simulink model "SCARA"  (R2015a)
settings: Solver=ode1  StartTime=0.0  StopTime=Inf  FixedStep=0.001  RelTol=1e-3
PostLoadFcn:
  | , if any(exist('dsrtsu_mdlpostloadfcn', 'file') == [2, 3, 6]), try dsrtsu_mdlpostloadfcn('Execute', bdroot); catch fprintf('Error in PostLoadFcn (dsrtsu_mdlpostloadfcn) for model "%s":\n %s\n', bdroot, lasterr); end, end,
libraries: rtilib1104 x9
settings Model: DSRTSU_INTERNAL_RTI_VER=460  DSRTSU_INTERNAL_RTI_TYPE=rti1104  DSRTSU_INTERNAL_RTIFPGA=50  CovHtmlReporting=off  Creator=k21s1315a  LastModifiedBy=k21s1315a
settings OptimizationCC: BlockReduction=off  OptimizeBlockIOStorage=off  BufferReuse=off  GlobalBufferReuse=off  ExpressionFolding=off  LocalBlockOutputs=off
settings HardwareCC: ProdIntDivRoundTo=Zero  ProdEndianess=BigEndian  ProdHWDeviceType=Generic->Custom  TargetIntDivRoundTo=Zero  TargetEndianess=BigEndian  TargetHWDeviceType=Generic->Custom
settings RTWCC: SystemTargetFile=rti1104.tlc  MakeCommand=make_rti  TemplateMakefile=rti1104.tmf  Description=dSPACE DS1104 Hardware Platform
settings STFCustomTargetCC: GenerateSampleERTMain=off  ParMdlRefBuildCompliant=on  GeneratePreprocessorConditionals=Disable all  ERTCustomFileBanners=off  SupportNonInlinedSFcns=on  SupportVariableSizeSignals=off  MATLABClassNameForMDSCustomization=Simulink.SoftwareTarget.GRTCustomization  GRTInterface=on  SystemTargetFile=rti1104.tlc
settings GRTTargetCC: CompOptLevelCompliant=off  ConcurrentExecutionCompliant=off  CombineOutputUpdateFcns=off  MatFileLogging=off  CPPClassGenCompliant=off  GRTInterface=on  ExtModeMexFile=noextcomm

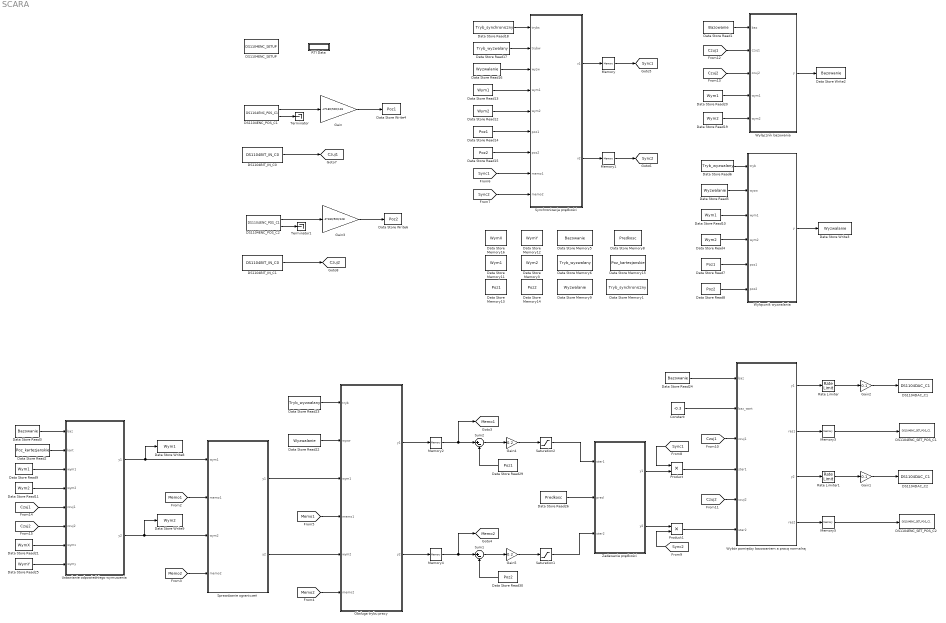
== system SCARA ==
  Constant : Constant  Value=-0.3
  DS1104BIT_IN_C0 : rtilib1104/DS1104 MASTER PPC/DS1104BIT_IN_C0  ChannelNo=0  Reserved1=[]  Reserved2=[]  Reserved3=[]  Reserved4=[]  DialogFcn=gui1104bit_in  UnitName={'DS1104BIT_IN_C'}  UnitValues={ 0 }  DSProperties=struct('RTI',struct('Version',uint32(1),'BlockType',struct('isSLSource',uint8(1),'isSLSink',uint8(0),'isHWSource',uint8(1),'isHWSink',uint8(0),'isSetup',uint8(0),'isInline',uint8(1),'isNonInline',uint8(0),'isInterrupt',uint8(0),'isChannelwise',uint8(1)),'IOBoardType','DS1104MASTER','UnitType','BIT','Identifier','BITINCH','DialogType','ML','BlockSet','NONE','SlaveProcessor','NONE'))
  DS1104BIT_IN_C1 : rtilib1104/DS1104 MASTER PPC/DS1104BIT_IN_C0  ChannelNo=1  Reserved1=[]  Reserved2=[]  Reserved3=[]  Reserved4=[]  DialogFcn=gui1104bit_in  UnitName={'DS1104BIT_IN_C'}  UnitValues={1}  DSProperties=struct('RTI',struct('Version',uint32(1),'BlockType',struct('isSLSource',uint8(1),'isSLSink',uint8(0),'isHWSource',uint8(1),'isHWSink',uint8(0),'isSetup',uint8(0),'isInline',uint8(1),'isNonInline',uint8(0),'isInterrupt',uint8(0),'isChannelwise',uint8(1)),'IOBoardType','DS1104MASTER','UnitType','BIT','Identifier','BITINCH','DialogType','ML','BlockSet','NONE','SlaveProcessor','NONE'))
  DS1104DAC_C1 : rtilib1104/DS1104 MASTER PPC/DS1104DAC_C1  ChannelNo=1  InitValue=0  TermMode=0  TermValue=0  Reserved1=[]  Reserved2=[]  Reserved3=[]  Reserved4=[]  DialogFcn=gui1104dac  UnitName={ 'DS1104DAC_C'}  UnitValues={ 1 }  DSProperties=struct('RTI',struct('Version',uint32(1),'BlockType',struct('isSLSource',uint8(0),'isSLSink',uint8(1),'isHWSource',uint8(0),'isHWSink',uint8(1),'isSetup',uint8(0),'isInline',uint8(1),'isNonInline',uint8(0),'isInterrupt',uint8(0),'isChannelwise',uint8(1)),'IOBoardType','DS1104MASTER','UnitType','DAC','Identifier','DAC','DialogType','ML','BlockSet','NONE','SlaveProcessor','NONE'))
  DS1104DAC_C2 : rtilib1104/DS1104 MASTER PPC/DS1104DAC_C1  ChannelNo=2  InitValue=0  TermMode=0  TermValue=0  Reserved1=[]  Reserved2=[]  Reserved3=[]  Reserved4=[]  DialogFcn=gui1104dac  UnitName={ 'DS1104DAC_C'}  UnitValues={2}  DSProperties=struct('RTI',struct('Version',uint32(1),'BlockType',struct('isSLSource',uint8(0),'isSLSink',uint8(1),'isHWSource',uint8(0),'isHWSink',uint8(1),'isSetup',uint8(0),'isInline',uint8(1),'isNonInline',uint8(0),'isInterrupt',uint8(0),'isChannelwise',uint8(1)),'IOBoardType','DS1104MASTER','UnitType','DAC','Identifier','DAC','DialogType','ML','BlockSet','NONE','SlaveProcessor','NONE'))
  DS1104ENC_POS_C1 : rtilib1104/DS1104 MASTER PPC/DS1104ENC_POS_C1  ChannelNo=1  PosValue=0  Reserved1=[]  Reserved2=[]  Reserved3=[]  Reserved4=[]  DialogFcn=gui1104enc_pos  UnitName={'DS1104ENC_POS_C'}  UnitValues={ 1 }  DSProperties=struct('RTI',struct('Version',uint32(1),'BlockType',struct('isSLSource',uint8(1),'isSLSink',uint8(0),'isHWSource',uint8(1),'isHWSink',uint8(0),'isSetup',uint8(0),'isInline',uint8(1),'isNonInline',uint8(0),'isInterrupt',uint8(0),'isChannelwise',uint8(1)),'IOBoardType','DS1104MASTER','UnitType','ENC','Identifier','ENCPOSCH','DialogType','ML','BlockSet','NONE','SlaveProcessor','NONE'))
  DS1104ENC_POS_C2 : rtilib1104/DS1104 MASTER PPC/DS1104ENC_POS_C1  ChannelNo=2  PosValue=0  Reserved1=[]  Reserved2=[]  Reserved3=[]  Reserved4=[]  DialogFcn=gui1104enc_pos  UnitName={'DS1104ENC_POS_C'}  UnitValues={2}  DSProperties=struct('RTI',struct('Version',uint32(1),'BlockType',struct('isSLSource',uint8(1),'isSLSink',uint8(0),'isHWSource',uint8(1),'isHWSink',uint8(0),'isSetup',uint8(0),'isInline',uint8(1),'isNonInline',uint8(0),'isInterrupt',uint8(0),'isChannelwise',uint8(1)),'IOBoardType','DS1104MASTER','UnitType','ENC','Identifier','ENCPOSCH','DialogType','ML','BlockSet','NONE','SlaveProcessor','NONE'))
  DS1104ENC_SETUP : rtilib1104/DS1104 MASTER PPC/DS1104ENC_SETUP  Reserved1=[]  Reserved2=[]  Reserved3=[]  Reserved4=[]  DialogFcn=gui1104enc_setup  UnitName={'DS1104ENC_SETUP'}  UnitValues={ [] }  DSProperties=struct('RTI',struct('Version',uint32(1),'BlockType',struct('isSLSource',uint8(0),'isSLSink',uint8(0),'isHWSource',uint8(0),'isHWSink',uint8(0),'isSetup',uint8(0),'isInline',uint8(1),'isNonInline',uint8(0),'isInterrupt',uint8(0),'isChannelwise',uint8(0)),'IOBoardType','DS1104MASTER','UnitType','ENC','Identifier','ENCSETUP','DialogType','ML','BlockSet','NONE','SlaveProcessor','NONE'))
      settings: SignalType=[0 0]
  DS1104ENC_SET_POS_C1 : rtilib1104/DS1104 MASTER PPC/DS1104ENC_SET_POS_C1  ChannelNo=1  PosValue=0  Reserved1=[]  Reserved2=[]  Reserved3=[]  Reserved4=[]  DialogFcn=gui1104enc_set_pos  UnitName={'DS1104ENC_SET_POS_C'}  UnitValues={ 1 }  DSProperties=struct('RTI',struct('Version',uint32(1),'BlockType',struct('isSLSource',uint8(0),'isSLSink',uint8(1),'isHWSource',uint8(0),'isHWSink',uint8(1),'isSetup',uint8(0),'isInline',uint8(1),'isNonInline',uint8(0),'isInterrupt',uint8(0),'isChannelwise',uint8(1)),'IOBoardType','DS1104MASTER','UnitType','ENC','Identifier','ENCRESET','DialogType','ML','BlockSet','NONE','SlaveProcessor','NONE'))
  DS1104ENC_SET_POS_C2 : rtilib1104/DS1104 MASTER PPC/DS1104ENC_SET_POS_C1  ChannelNo=2  PosValue=0  Reserved1=[]  Reserved2=[]  Reserved3=[]  Reserved4=[]  DialogFcn=gui1104enc_set_pos  UnitName={'DS1104ENC_SET_POS_C'}  UnitValues={2}  DSProperties=struct('RTI',struct('Version',uint32(1),'BlockType',struct('isSLSource',uint8(0),'isSLSink',uint8(1),'isHWSource',uint8(0),'isHWSink',uint8(1),'isSetup',uint8(0),'isInline',uint8(1),'isNonInline',uint8(0),'isInterrupt',uint8(0),'isChannelwise',uint8(1)),'IOBoardType','DS1104MASTER','UnitType','ENC','Identifier','ENCRESET','DialogType','ML','BlockSet','NONE','SlaveProcessor','NONE'))
  Data Store Memory1 : DataStoreMemory  DataStoreName=Tryb_synchroniczny  ReadBeforeWriteMsg=warning  WriteAfterWriteMsg=warning  WriteAfterReadMsg=warning
  Data Store Memory11 : DataStoreMemory  DataStoreName=Wym1  ReadBeforeWriteMsg=warning  WriteAfterWriteMsg=warning  WriteAfterReadMsg=warning
  Data Store Memory12 : DataStoreMemory  DataStoreName=WymY  ReadBeforeWriteMsg=warning  WriteAfterWriteMsg=warning  WriteAfterReadMsg=warning
  Data Store Memory13 : DataStoreMemory  DataStoreName=Poz1  ReadBeforeWriteMsg=warning  WriteAfterWriteMsg=warning  WriteAfterReadMsg=warning
  Data Store Memory14 : DataStoreMemory  DataStoreName=Poz2  ReadBeforeWriteMsg=warning  WriteAfterWriteMsg=warning  WriteAfterReadMsg=warning
  Data Store Memory15 : DataStoreMemory  DataStoreName=Poz_kartezjanskie  ReadBeforeWriteMsg=warning  WriteAfterWriteMsg=warning  WriteAfterReadMsg=warning
  Data Store Memory16 : DataStoreMemory  DataStoreName=WymX  ReadBeforeWriteMsg=warning  WriteAfterWriteMsg=warning  WriteAfterReadMsg=warning
  Data Store Memory3 : DataStoreMemory  DataStoreName=Wym2  ReadBeforeWriteMsg=warning  WriteAfterWriteMsg=warning  WriteAfterReadMsg=warning
  Data Store Memory5 : DataStoreMemory  DataStoreName=Bazowanie  ReadBeforeWriteMsg=warning  WriteAfterWriteMsg=warning  WriteAfterReadMsg=warning
  Data Store Memory6 : DataStoreMemory  DataStoreName=Tryb_wyzwalany  ReadBeforeWriteMsg=warning  WriteAfterWriteMsg=warning  WriteAfterReadMsg=warning
  Data Store Memory8 : DataStoreMemory  DataStoreName=Predkosc  ReadBeforeWriteMsg=warning  WriteAfterWriteMsg=warning  WriteAfterReadMsg=warning
  Data Store Memory9 : DataStoreMemory  DataStoreName=Wyzwalanie  ReadBeforeWriteMsg=warning  WriteAfterWriteMsg=warning  WriteAfterReadMsg=warning
  Data Store Read1 : DataStoreRead  DataStoreName=Bazowanie
  Data Store Read{9..10,13,20} (4 alike) : DataStoreRead  DataStoreName=Wym1
  Data Store Read{4,11..12,19} (4 alike) : DataStoreRead  DataStoreName=Wym2
  Data Store Read14 : DataStoreRead  DataStoreName=Poz1
  Data Store Read15 : DataStoreRead  DataStoreName=Poz2
  Data Store Read16 : DataStoreRead  DataStoreName=Wyzwalanie
  Data Store Read17 : DataStoreRead  DataStoreName=Tryb_wyzwalany
  Data Store Read18 : DataStoreRead  DataStoreName=Tryb_synchroniczny
  Data Store Read2 : DataStoreRead  DataStoreName=Poz_kartezjanskie
  Data Store Read21 : DataStoreRead  DataStoreName=WymX
  Data Store Read22 : DataStoreRead  DataStoreName=Wyzwalanie
  Data Store Read23 : DataStoreRead  DataStoreName=Tryb_wyzwalany
  Data Store Read24 : DataStoreRead  DataStoreName=Bazowanie
  Data Store Read25 : DataStoreRead  DataStoreName=WymY
  Data Store Read26 : DataStoreRead  DataStoreName=Predkosc
  Data Store Read29 : DataStoreRead  DataStoreName=Poz1
  Data Store Read3 : DataStoreRead  DataStoreName=Bazowanie
  Data Store Read30 : DataStoreRead  DataStoreName=Poz2
  Data Store Read5 : DataStoreRead  DataStoreName=Wyzwalanie
  Data Store Read6 : DataStoreRead  DataStoreName=Tryb_wyzwalany
  Data Store Read7 : DataStoreRead  DataStoreName=Poz1
  Data Store Read8 : DataStoreRead  DataStoreName=Poz2
  Data Store Write2 : DataStoreWrite  DataStoreName=Bazowanie
  Data Store Write3 : DataStoreWrite  DataStoreName=Wyzwalanie
  Data Store Write4 : DataStoreWrite  DataStoreName=Poz1
  Data Store Write6 : DataStoreWrite  DataStoreName=Poz2
  Data Store Write8 : DataStoreWrite  DataStoreName=Wym1
  Data Store Write9 : DataStoreWrite  DataStoreName=Wym2
  Gain : Gain  Gain=-2*180/500/128
  Gain1 : Gain  Gain=0.1
  Gain2 : Gain  Gain=0.1
  Gain3 : Gain  Gain=-2*180/500/128
  Gain4 : Gain  Gain=0.2
  Gain5 : Gain  Gain=0.2
  Memory{,1,3,5} (4 alike) : Memory  X0=1
  Memory2 : Memory
  Memory4 : Memory
  Obsługa trybu pracy : MATLAB Function  TreatAsAtomicUnit=on
  Product : Product
  Product1 : Product
  RTI Data : Subsystem  Tag=struct('RTIDataServer',struct('RTIDataServerVs','2','RTIModelDescription','struct(''main'',''Scara_model'',''sub'','''',''isMp'',0)'))  LoadFcn="if exist('rtidc'), try,  rtidc('DataHostBlockClbLoad', gcbh); catch, disp(['Warning: ''LoadFcn'' for RTI Data block failed: ' lasterr]); end, end,"  mask(RTI_DATA_HOST){}
      mask help:
      | RTI Data Block.
      | This block is used by RTI to store internal model-dependent data.
      | Please keep this block on the root level of the model. Deleting this block will result in data loss.
      |
      | NEVER DELETE OR COPY THIS BLOCK!
      settings: CopyFcn="if exist('rtidc'), try,  rtidc('DataHostBlockClbCopy', gcbh); catch, disp(['Warning: ''CopyFcn'' for RTI Data block failed: ' lasterr]); end, end,"  DeleteFcn="if exist('rtidc'), try,  rtidc('DataHostBlockClbDelete', gcbh); catch, disp(['Warning: ''DeleteFcn'' for RTI Data block failed: ' lasterr]); end, end,"  ModelCloseFcn="if exist('rtidc'), try,  rtidc('DataHostBlockClbModelClose', gcbh); catch, disp(['Warning: ''ModelCloseFcn'' for RTI Data block failed: ' lasterr]); end, end,"  PreSaveFcn="if exist('rtidc'), try,  rtidc('DataHostBlockClbPreSave', gcbh); catch, disp(['Warning: ''PreSaveFcn'' for RTI Data block failed: ' lasterr]); end, end,"  PostSaveFcn="if exist('rtidc'), try,  rtidc('DataHostBlockClbPostSave', gcbh); catch, disp(['Warning: ''PostSaveFcn'' for RTI Data block failed: ' lasterr]); end, end,"  NameChangeFcn="if exist('rtidc'), try,  rtidc('DataHostBlockClbNameChange', gcbh); catch, disp(['Warning: ''NameChangeFcn'' for RTI Data block failed: ' lasterr]); end, end,"
      mask Help:
      | RTI Data Block.
      | This block is used by RTI to store internal model-dependent data.
      | Please keep this block on the root level of the model. Deleting this block will result in data loss.
      | 
      | NEVER DELETE OR COPY THIS BLOCK!
      mask Display:
      | text(0.5, 0.5, 'RTI Data', 'HorizontalAlignment', 'center');
      | plot([1 0]);
  Rate Limiter : RateLimiter  RisingSlewLimit=50  FallingSlewLimit=-50  SampleTimeMode=inherited
  Rate Limiter1 : RateLimiter  RisingSlewLimit=50  FallingSlewLimit=-50  SampleTimeMode=inherited
  Saturation1 : Saturate  UpperLimit=3  LowerLimit=-3
  Saturation2 : Saturate  UpperLimit=3  LowerLimit=-3
  Sprawdzanie ograniczeń : MATLAB Function  TreatAsAtomicUnit=on
  Sum1 : Sum  Inputs=|+-
  Sum2 : Sum  Inputs=|+-
  Synchronizacja prędkości : MATLAB Function  TreatAsAtomicUnit=on
  Terminator : Terminator
  Terminator1 : Terminator
  "Ustawianie odpowiedniego wymuszenia " : MATLAB Function  TreatAsAtomicUnit=on
  Wybór pomiędzy bazowaniem a pracą normalną : MATLAB Function  TreatAsAtomicUnit=on
  Wyłącznik bazowania : MATLAB Function  TreatAsAtomicUnit=on
  "Wyłącznik wyzwalania " : MATLAB Function  TreatAsAtomicUnit=on
  Zadawanie prędkości : MATLAB Function  TreatAsAtomicUnit=on
  tag scope: Czuj1=global, Czuj2=global, Memo1=global, Memo2=global, Sync1=global, Sync2=global
  wires:
  DS1104ENC_POS_C1/2 -> Terminator/1
  DS1104ENC_POS_C1/1 -> Gain/1
  DS1104ENC_POS_C2/2 -> Terminator1/1
  DS1104ENC_POS_C2/1 -> Gain3/1
  Rate Limiter/1 -> Gain2/1
  Gain2/1 -> DS1104DAC_C1/1
  DS1104BIT_IN_C0/1 -> [Czuj1]
  DS1104BIT_IN_C1/1 -> [Czuj2]
  Data Store Read19/1 -> Wyłącznik bazowania/5(wym2)
  Data Store Read20/1 -> Wyłącznik bazowania/4(wym1)
  [Czuj2] -> Wyłącznik bazowania/3(czuj2)
  [Czuj1] -> Wyłącznik bazowania/2(czuj1)
  Data Store Read1/1 -> Wyłącznik bazowania/1(baz)
  Wyłącznik bazowania/1(y) -> Data Store Write2/1
  Data Store Read5/1 -> "Wyłącznik wyzwalania "/2(wyzw)
  Data Store Read6/1 -> "Wyłącznik wyzwalania "/1(tryb)
  Data Store Read10/1 -> "Wyłącznik wyzwalania "/3(wym1)
  Data Store Read4/1 -> "Wyłącznik wyzwalania "/4(wym2)
  Gain3/1 -> Data Store Write6/1
  Data Store Read7/1 -> "Wyłącznik wyzwalania "/5(poz1)
  Data Store Read8/1 -> "Wyłącznik wyzwalania "/6(poz2)
  "Wyłącznik wyzwalania "/1(y) -> Data Store Write3/1
  Gain/1 -> Data Store Write4/1
  Data Store Read13/1 -> Synchronizacja prędkości/4(wym1)
  Data Store Read12/1 -> Synchronizacja prędkości/5(wym2)
  Data Store Read14/1 -> Synchronizacja prędkości/6(poz1)
  Data Store Read15/1 -> Synchronizacja prędkości/7(poz2)
  Data Store Read16/1 -> Synchronizacja prędkości/3(wyzw)
  Data Store Read17/1 -> Synchronizacja prędkości/2(trybw)
  Data Store Read18/1 -> Synchronizacja prędkości/1(trybs)
  [Sync2] -> Synchronizacja prędkości/9(memo2)
  [Sync1] -> Synchronizacja prędkości/8(memo1)
  Synchronizacja prędkości/1(v1) -> Memory/1
  Memory/1 -> [Sync1]
  Synchronizacja prędkości/2(v2) -> Memory1/1
  Memory1/1 -> [Sync2]
  "Ustawianie odpowiedniego wymuszenia "/1(y1) -> Data Store Write8/1, Sprawdzanie ograniczeń/1(wym1)
  "Ustawianie odpowiedniego wymuszenia "/2(y2) -> Data Store Write9/1, Sprawdzanie ograniczeń/3(wym2)
  Sprawdzanie ograniczeń/2(y2) -> Obsługa trybu pracy/5(wym2)
  Sprawdzanie ograniczeń/1(y1) -> Obsługa trybu pracy/3(wym1)
  [Memo1] -> Sprawdzanie ograniczeń/2(memo1)
  [Memo2] -> Sprawdzanie ograniczeń/4(memo2)
  [Memo2] -> Obsługa trybu pracy/6(memo2)
  [Memo1] -> Obsługa trybu pracy/4(memo1)
  Data Store Read22/1 -> Obsługa trybu pracy/2(wyzw)
  Data Store Read23/1 -> Obsługa trybu pracy/1(tryb)
  Data Store Read26/1 -> Zadawanie prędkości/2(pred)
  Saturation2/1 -> Zadawanie prędkości/1(ster1)
  Data Store Read24/1 -> Wybór pomiędzy bazowaniem a pracą normalną/1(baz)
  Memory3/1 -> DS1104ENC_SET_POS_C1/Trigger
  Wybór pomiędzy bazowaniem a pracą normalną/1(y1) -> Rate Limiter/1
  Constant/1 -> Wybór pomiędzy bazowaniem a pracą normalną/2(baz_wart)
  Wybór pomiędzy bazowaniem a pracą normalną/2(res1) -> Memory3/1
  Gain5/1 -> Saturation1/1
  Data Store Read30/1 -> Sum1/2
  Obsługa trybu pracy/2(y2) -> Memory4/1
  Sum1/1 -> Gain5/1
  Memory4/1 -> [Memo2], Sum1/1
  Saturation1/1 -> Zadawanie prędkości/3(ster2)
  Data Store Read29/1 -> Sum2/2
  Memory2/1 -> [Memo1], Sum2/1
  Sum2/1 -> Gain4/1
  Gain4/1 -> Saturation2/1
  Obsługa trybu pracy/1(y1) -> Memory2/1
  [Sync2] -> Product1/2
  Zadawanie prędkości/2(y2) -> Product1/1
  [Sync1] -> Product/1
  Zadawanie prędkości/1(y1) -> Product/2
  Product/1 -> Wybór pomiędzy bazowaniem a pracą normalną/4(ster1)
  Product1/1 -> Wybór pomiędzy bazowaniem a pracą normalną/6(ster2)
  [Czuj1] -> Wybór pomiędzy bazowaniem a pracą normalną/3(czuj1)
  [Czuj2] -> Wybór pomiędzy bazowaniem a pracą normalną/5(czuj2)
  Data Store Read3/1 -> "Ustawianie odpowiedniego wymuszenia "/1(baz)
  Data Store Read2/1 -> "Ustawianie odpowiedniego wymuszenia "/2(kart)
  Data Store Read9/1 -> "Ustawianie odpowiedniego wymuszenia "/3(wym1)
  Data Store Read11/1 -> "Ustawianie odpowiedniego wymuszenia "/4(wym2)
  Data Store Read21/1 -> "Ustawianie odpowiedniego wymuszenia "/7(wymx)
  Data Store Read25/1 -> "Ustawianie odpowiedniego wymuszenia "/8(wymy)
  Memory5/1 -> DS1104ENC_SET_POS_C2/Trigger
  Wybór pomiędzy bazowaniem a pracą normalną/4(res2) -> Memory5/1
  Wybór pomiędzy bazowaniem a pracą normalną/3(y2) -> Rate Limiter1/1
  [Czuj1] -> "Ustawianie odpowiedniego wymuszenia "/5(czuj1)
  [Czuj2] -> "Ustawianie odpowiedniego wymuszenia "/6(czuj2)
  Rate Limiter1/1 -> Gain1/1
  Gain1/1 -> DS1104DAC_C2/1

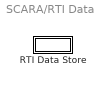
== system SCARA/RTI Data ==
  RTI Data Store : Subsystem  Tag="struct('private',struct('version',struct('dsVer',uint32(2),'dsVerCreation',uint32(2),'RTI',struct('ver','7.4','type','RTI1104')),'access',struct('type','Model','isPerm',1,'created',['08-Dec-2021 13:39:11'],'modified',['15-Dec-2021 14:24:32'],'location','')),'public',struct('main',struct('data',[]),'sub',struct('name',{{'Scara_model'}},'data',{{struct('TH',struct('thTaskInfo',struct('taskType',{'TIMER','HWINT','TMRINT','SWINT','GLINT'},'tasksNumOf',{1,0,0,0,0},'srcIds',{{'TIMERA'},{},{},{},{}},'taskNames',{{['Timer Task 1']},{},{},{},{}})),'th_tc',struct('dataType','TASK','taskGroupId','','taskGroupList',{{}},'taskSchedulingPolicy','FCFS','taskType','TIMER','blkh',-1,'srcId','TIMERA','srcSgnName',['Timer A interrupt'],'srcCpuName','','taskName',['Timer Task 1  [0.001] s'],'taskNameDisplayExt','','smplTime',0.001,'smplTimeOffs',0,'hasFixedPriority',0,'priority',1,'hasFixedOvc',0,'ovcType',1,'ovcMax',1),'tc_th',struct('dataType','TASK','taskGroupId','','taskGroupList',{{}},'taskSchedulingPolicy','FCFS','taskType','TIMER','blkh',-1,'srcId','TIMERA','srcSgnName',['Timer A interrupt'],'srcCpuName','','taskName',['Timer Task 1  [0.001] s'],'taskNameDisplayExt','','smplTime',0.001,'smplTimeOffs',0,'hasFixedPriority',0,'priority',1,'hasFixedOvc',0,'ovcType',1,'ovcMax',1))}})))"  mask(RTI_DATA_STORE){}
      mask help:
      | RTI Data Store Block. This block is used by RTI to store internal model dependent data. Deleting this block will result in data loss.
      |
      | NEVER DELETE, COPY, OR MODIFY THIS BLOCK!
      mask Help:
      | RTI Data Store Block. This block is used by RTI to store internal model dependent data. Deleting this block will result in data loss.
      | 
      | NEVER DELETE, COPY, OR MODIFY THIS BLOCK!
      mask Display: text(0.5, 0.5, ' ', 'HorizontalAlignment', 'center');

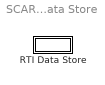
== system SCARA/RTI Data/RTI Data Store ==
  RTI Data Store : Subsystem  mask(RTI_DATA_STORE){}
      mask help:
      | RTI Data Store Block. This block is used by RTI to store internal model dependent data. Deleting this block will result in data loss.
      |
      | NEVER DELETE, COPY, OR MODIFY THIS BLOCK!
      mask Help:
      | RTI Data Store Block. This block is used by RTI to store internal model dependent data. Deleting this block will result in data loss.
      | 
      | NEVER DELETE, COPY, OR MODIFY THIS BLOCK!
      mask Display: text(0.5, 0.5, ' ', 'HorizontalAlignment', 'center');

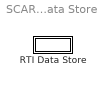
== system SCARA/RTI Data/RTI Data Store/RTI Data Store ==
  RTI Data Store : Subsystem  mask(RTI_DATA_STORE){}
      mask help:
      | RTI Data Store Block. This block is used by RTI to store internal model dependent data. Deleting this block will result in data loss.
      |
      | NEVER DELETE, COPY, OR MODIFY THIS BLOCK!
      mask Help:
      | RTI Data Store Block. This block is used by RTI to store internal model dependent data. Deleting this block will result in data loss.
      | 
      | NEVER DELETE, COPY, OR MODIFY THIS BLOCK!
      mask Display: text(0.5, 0.5, ' ', 'HorizontalAlignment', 'center');

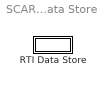
== system SCARA/RTI Data/RTI Data Store/RTI Data Store/RTI Data Store ==
  RTI Data Store : Subsystem  mask(RTI_DATA_STORE){}
      mask help:
      | RTI Data Store Block. This block is used by RTI to store internal model dependent data. Deleting this block will result in data loss.
      |
      | NEVER DELETE, COPY, OR MODIFY THIS BLOCK!
      mask Help:
      | RTI Data Store Block. This block is used by RTI to store internal model dependent data. Deleting this block will result in data loss.
      | 
      | NEVER DELETE, COPY, OR MODIFY THIS BLOCK!
      mask Display: text(0.5, 0.5, ' ', 'HorizontalAlignment', 'center');

== system SCARA/RTI Data/RTI Data Store/RTI Data Store/RTI Data Store/RTI Data Store ==

== matlab function SCARA/Wyłącznik bazowania ==
  data: baz input; czuj1 input; y output; czuj2 input; wym1 input; wym2 input
function y = fcn(baz, czuj1, czuj2, wym1, wym2)
if baz && ~czuj1 && ~czuj2 && ~wym1 && ~wym2
    y = 0;
else
    y = baz;
end

== matlab function SCARA/Wyłącznik wyzwalania  ==
  data: tryb input; wyzw input; wym1 input; wym2 input; y output; poz1 input; poz2 input
function y = fcn(tryb, wyzw, wym1, wym2, poz1, poz2)
eps = 1;
if tryb && wyzw && abs(wym1-poz1) <= eps && abs(wym2-poz2) <= eps
    y = 0;
else
    y = wyzw;
end

== matlab function SCARA/Synchronizacja prędkości ==
  data: trybs input; trybw input; v1 output; wyzw input; wym1 input; wym2 input; poz1 input; poz2 input; memo1 input; memo2 input; v2 output
function [v1, v2] = fcn(trybs, trybw, wyzw, wym1, wym2, poz1, poz2, memo1, memo2)
% Wyliczanie synchronizacji prędkości przed wyzwoleniem
if trybs && trybw && ~wyzw
    angle1 = abs(wym1-poz1);
    angle2 = abs(wym2-poz2);
    if angle1 >= angle2
        v1 = 1;
        v2 = angle2/angle1;
    else
        v1 = angle1/angle2;
        v2 = 1;
    end
% Podtrzymanie wyliczonych prędkości po wyzwoleniu
elseif trybs && trybw && wyzw
    v1 = memo1;
    v2 = memo2;
% Nieuwzględnianie synchronizacji przy trybie "pracy ręcznej" oraz przy
% wyłączonym trybie PTP Synchronicznym
else
    v1 = 1;
    v2 = 1;
end

== matlab function SCARA/Ustawianie odpowiedniego wymuszenia  ==
  data: baz input; kart input; y1 output; wym1 input; wym2 input; czuj1 input; czuj2 input; wymx input; wymy input; y2 output
function [y1, y2] = fcn(baz, kart, wym1, wym2, czuj1, czuj2, wymx, wymy)
% Długości ramion robota w milimetrach [mm]
a1 = 630;
a2 = 510;
% Wyliczanie potrzebnych danych do odwrotnej kinematyki
cosphi2 = (a1^2 + a2^2 - wymx^2 - wymy^2) / (2 * a1 * a2);
sinphi2 = (1 - cosphi2^2)^0.5;
phi1 = atan2(sinphi2, cosphi2);
phi2 = atan2(wymy, wymx) - atan2(a2 * sinphi2, a1 - a2 * cosphi2);
% Wymuszenie 1
if baz && ~czuj1
    y1 = 0;
elseif kart
    y1 = phi2 * 180 / pi;
else
    y1 = wym1;
end
% Wymuszenie 2
if baz && ~czuj2
    y2 = 0;
elseif kart
    y2 = phi1 * 180 / pi;
else
    y2 = wym2;
end

== matlab function SCARA/Sprawdzanie ograniczeń ==
  data: wym1 input; y1 output; memo1 input; wym2 input; memo2 input; y2 output
function [y1, y2] = fcn(wym1, memo1, wym2, memo2)
if wym1 < -180 || wym1 > 180 || wym2 <-180 || wym2 > 180
    y1 = memo1;
    y2 = memo2;
else
    y1 = wym1;
    y2 = wym2;
end

== matlab function SCARA/Wybór pomiędzy bazowaniem a pracą normalną ==
  data: baz input; baz_wart input; czuj1 input; ster1 input; czuj2 input; y1 output; res1 output; y2 output; res2 output; ster2 input
function [y1, res1, y2, res2] = fcn(baz, baz_wart, czuj1, ster1, czuj2, ster2)
% Sterowanie 1
if baz && czuj1
    y1 = baz_wart;
    res1 = 0;
elseif baz && ~czuj1 && czuj2 
   y1 = 0;
   res1 = 0;
else
    y1 = ster1;
    res1 = 1;
end
% Sterowanie 2
if baz && ~czuj1 && czuj2
    y2 = baz_wart;
    res2 = 0;
elseif baz && czuj1
    y2 = 0;
    res2 = 0;
else
    y2 = ster2;
    res2 = 1;
end

== matlab function SCARA/Obsługa trybu pracy ==
  data: tryb input; y1 output; wyzw input; wym1 input; memo1 input; wym2 input; memo2 input; y2 output
function [y1, y2] = fcn(tryb, wyzw, wym1, memo1, wym2, memo2)
% Tryb "pracy ręcznej"
if ~tryb
    y1 = wym1;
    y2 = wym2;
% Tryb "wyzwalany"
else
    if ~wyzw
        y1 = memo1;
        y2 = memo2;
    else
        y1 = wym1;
        y2 = wym2;
    end
end

== matlab function SCARA/Zadawanie prędkości ==
  data: ster1 input; pred input; ster2 input; y1 output; y2 output
function [y1, y2] = fcn(ster1, pred, ster2)
if pred >= 1 && pred <= 100
    y1 = ster1*pred/100;
    y2 = ster2*pred/100;
else
    y1 = ster1;
    y2 = ster2;
end
